simulink model "Bordes"  (R2022a)
settings: Solver=VariableStepAuto  StartTime=0.0  StopTime=inf  RelTol=1e-3
undefined symbols (not defined in the file or in its folder): none, videoinput
libraries: imaqlib x1, visionconversions x1
settings Model: Creator=jonathan  LastModifiedBy=jonathan

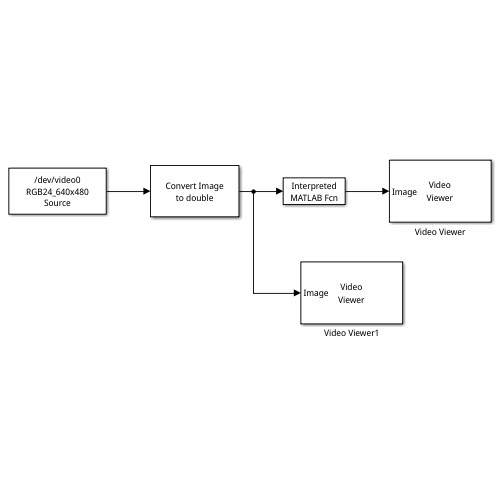
[thumbnail: Simulink's stored preview of the top-level diagram]
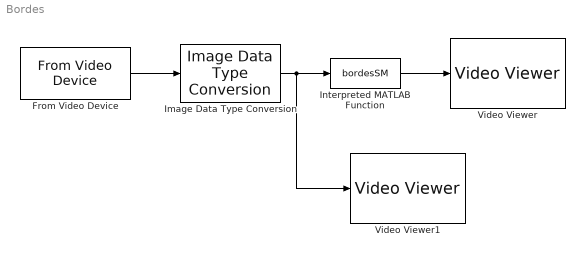
== system Bordes ==
  From Video Device : imaqlib/From Video Device  DeviceMenu=linuxvideo 1 (/dev/video0)  Device=linuxvideo 1 (/dev/video0)  ObjConstructor=videoinput('linuxvideo', 1)  VideoFormatMenu=RGB24_640x480  VideoFormat=RGB24_640x480  VideoSource=Source  ROIPosition=[0 0 480 640]  EnableHWTrigger=off  TriggerConfiguration=none/none  SampleTime=1/30  OutputPortsMode=One multidimensional signal  DataType=single  CanDoHWTrigger=no  ReturnedColorSpace=grayscale  BlockHandle=4.0002  ROIWidth=640  ROIHeight=480  ROIColumn=0  ROIRow=0  EngXMLPath=/usr/local/MATLAB/R2022a/toolbox/imaq/imaq/private  DevXMLPath=/home/jonathan/Documents/MATLAB/SupportPackages/R2022a/toolbox/imaq/supportpackages/genericvideo/adaptor/glnxa64  EngLibPath=/usr/local/MATLAB/R2022a/toolbox/imaq/imaqblks/imaqmex/glnxa64  ColorSpace=grayscale  BayerSensorAlignment=grbg  ImaqMode=off
  Image Data Type Conversion : visionconversions/Image Data Type Conversion  outDT=double  isSigned=on  wordLen=16  numFracBits=0
      settings: SourceProductBaseCode=VP
  Interpreted MATLAB Function : MATLABFcn  MATLABFcn=bordesSM  Output1D=off
  Video Viewer : VideoViewer  FigPos=[-76 929 1332 608]
  Video Viewer1 : VideoViewer  FigPos=[965 624 406 300]
  wires:
  From Video Device/1 -> Image Data Type Conversion/1
  Image Data Type Conversion/1 -> Video Viewer1/1, Interpreted MATLAB Function/1
  Interpreted MATLAB Function/1 -> Video Viewer/1
